simulink model "Li_Slotine"  (R2021b)
settings: Solver=VariableStepAuto  StartTime=0.0  StopTime=15.0  RelTol=1e1
values from neighbouring files (symbols this model uses):
  Kd = 100 * diag([1 5 3 1 1 1])    [GuadagniControllore.m]
  lambda = 1*diag([20 30 30 12 10 50])    [GuadagniControllore.m]
  m1 = L(1).m    [GuadagniControllore.m]
  m2 = L(2).m    [GuadagniControllore.m]
  m3 = L(3).m    [GuadagniControllore.m]
  m4 = L(4).m    [GuadagniControllore.m]
  m5 = L(5).m    [GuadagniControllore.m]
  m6 = L(6).m    [GuadagniControllore.m]
undefined symbols (not defined in the file or in its folder): B, l1, l2, l3, l4, l5, l6, r, Spline
libraries: roblocks x2, robotcorelib x1, simulink x1
(part 5 of 5)

== matlab function Li_Slotine/Li-Slotine control/parameters estimation ==
  data: Y input; dpi output; s input
function dpi = dyn_param(Y, s)
% Definisco una matrice definita positiva
R = 5*diag([0.1 11 25 54 55 298]);
% Calcolo la dinamica di stima dei parametri
dpi = inv(R) * Y' * s;

== matlab function Li_Slotine/Li-Slotine control/MATLAB Function ==
  data: e input; qr_d output; e_dot input; qd_des input; qdd_des input; qr_dd output; lambda input
function [qr_d, qr_dd] = qr_d_calculus(e, e_dot, qd_des, qdd_des, lambda)
% Calcolo qr_d
qr_d = qd_des + lambda*e;
% Calcolo qr_dd
qr_dd = qdd_des + lambda*e_dot;
